simulink model "M03_Cascaded_ActiveYaw"  (R2025b)
settings: Solver=VariableStepAuto  StartTime=0.0  StopTime=t_sim_stop  RelTol=1e-3
undefined symbols (not defined in the file): a, b, g, k, L, mass, mu, P_gains, path_waypoints, v_ref_array, Vx_breakpoints
libraries: simulink x2, autolibshared x1
settings Model: Creator=Legion  LastModifiedBy=Legion

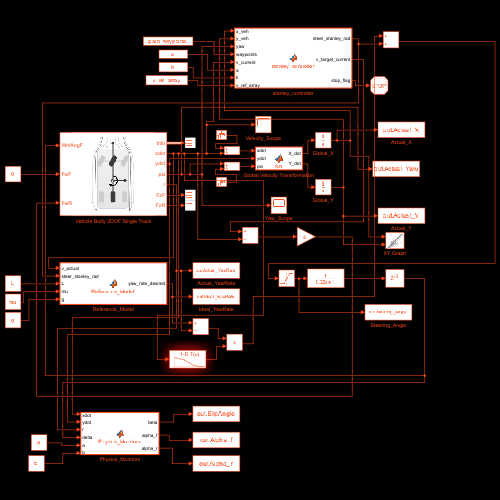
[thumbnail: Simulink's stored preview of the top-level diagram]
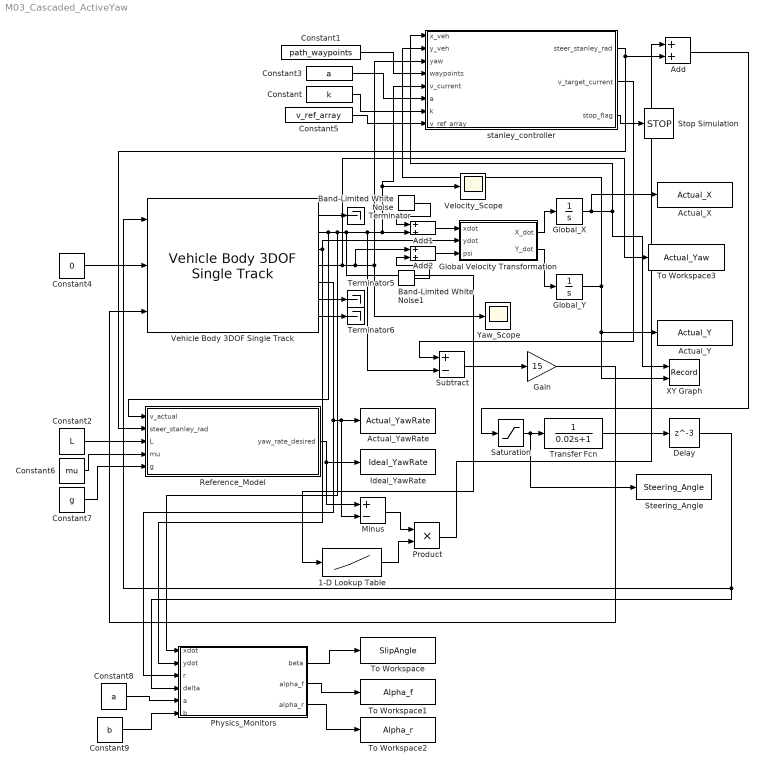
== system M03_Cascaded_ActiveYaw ==
  1-D Lookup Table : Lookup_n-D  NumberOfTableDimensions=1  BreakpointsForDimension1=Vx_breakpoints  Table=P_gains  InternalRulePriority=Speed  RndMeth=Simplest
  Actual_X : ToWorkspace  VariableName=Actual_X  SaveFormat=Timeseries  SampleTime=-1
  Actual_Y : ToWorkspace  VariableName=Actual_Y  SaveFormat=Timeseries  SampleTime=-1
  Actual_YawRate : ToWorkspace  VariableName=Actual_YawRate  SaveFormat=Timeseries  SampleTime=-1
  Add : Sum
  Add1 : Sum
  Add2 : Sum
  Band-Limited White Noise : simulink/Sources/Band-Limited White Noise  Cov=[0.0001]  Ts=0.01  seed=[23341]
  Band-Limited White Noise1 : simulink/Sources/Band-Limited White Noise  Cov=[0.0005]  Ts=0.01  seed=[23341]
  Constant : Constant  Value=k
  Constant1 : Constant  Value=path_waypoints
  Constant2 : Constant  Value=L
  Constant3 : Constant  Value=a
  Constant4 : Constant  Value=0
  Constant5 : Constant  Value=v_ref_array
  Constant6 : Constant  Value=mu
  Constant7 : Constant  Value=g
  Constant8 : Constant  Value=a
  Constant9 : Constant  Value=b
  Delay : Delay  DelayLength=3
  Gain : Gain  Gain=15
  Global Velocity Transformation : MATLAB Function  TreatAsAtomicUnit=on
  Global_X : Integrator  InitialCondition=path_waypoints(1,1)
  Global_Y : Integrator  InitialCondition=path_waypoints(1,2)
  Ideal_YawRate : ToWorkspace  VariableName=Ideal_YawRate  SaveFormat=Timeseries  SampleTime=-1
  Minus : Sum  Inputs=+-
  Physics_Monitors : MATLAB Function  TreatAsAtomicUnit=on
  Product : Product
  Reference_Model : MATLAB Function  TreatAsAtomicUnit=on
  Saturation : Saturate  UpperLimit=30 * pi/180  LowerLimit=-30 * pi/180
  Steering_Angle : ToWorkspace  VariableName=Steering_Angle  SaveFormat=Timeseries  SampleTime=-1
  Stop Simulation : Stop
  Subtract : Sum  Inputs=+-
  Terminator : Terminator
  Terminator5 : Terminator
  Terminator6 : Terminator
  To Workspace : ToWorkspace  VariableName=SlipAngle  SaveFormat=Timeseries  SampleTime=-1
  To Workspace1 : ToWorkspace  VariableName=Alpha_f  SaveFormat=Timeseries  SampleTime=-1
  To Workspace2 : ToWorkspace  VariableName=Alpha_r  SaveFormat=Timeseries  SampleTime=-1
  To Workspace3 : ToWorkspace  VariableName=Actual_Yaw  SaveFormat=Timeseries  SampleTime=-1
  Transfer Fcn : TransferFcn  Denominator=[0.02 1]
  Vehicle Body 3DOF Single Track : autolibshared/Vehicle Body 3DOF Single Track  trackMode=Single (bicycle)  inputMode=External longitudinal forces  frontSteerMode=on  rearSteerMode=off  windMode=off  muMode=off  extFMode=off  extMMode=off  htchFMode=off  htchMMode=off  extXo=off  extpsio=off  extxdoto=off  extro=off  extYo=off  extTamb=off  extydoto=off  aMode=2  NF=2  NR=2  m=mass  a=a  b=b  h=h  dh=1  hh=0.2  X_o=0  xdot_o=0.01  CalphaMode=off  sigmaMode=off  d=0  hl=0  w=[1.4,1.4]  Cy_f=Cy_f  Cy_r=Cy_r  sigma_f=.1  sigma_r=.1  alpha_f_brk=[-0.785, -0.628, -0.471, -0.314, -0.157, 0.000, 0.157, 0.314, 0.471, 0.628, 0.785]  Cy_f_data=[2000, 3000, 4000, 5500, 7000, 9000, 7000, 5500, 4000, 3000, 2000]  alpha_r_brk=[-0.785, -0.628, -0.471, -0.314, -0.157, 0.000, 0.157, 0.314, 0.471, 0.628, 0.785]  Cy_r_data=[2000, 3000, 4000, 5500, 7000, 9000, 7000, 5500, 4000, 3000, 2000]  Y_o=0  ydot_o=0  Izz=Izz  psi_o=atan2(path_waypoints(2,2)-path_waypoints(1,2), path_waypoints(2,1)-path_waypoints(1,1))  r_o=0  Af=Af  Cd=.3  Cl=.1  Cpm=.1  beta_w=[0 0.01:0.01:0.3]  Cs=[0 0.01:0.01:0.3]  Cym=[0 1e-6:0.01:0.3]  Pabs=101325  Tair=273  g=9.81  mu=mu  xdot_tol=.01  Fznom=Fznom  Fxtire_sat=7e4  Fytire_sat=7e4  longOff=0  latOff=0  vertOff=0  wrapAng=off
  Velocity_Scope : Scope
      settings: ActiveDisplayYMinimum=0.7024131164666485  ActiveDisplayYMaximum=1.4316639746586821
  XY Graph : Record  NumPorts=2.0  FileSettingsInternal="{\"entries\":[{\"content\":{\"excelSettings\":{\"content\":{},\"type\":\"Streamout.ExcelSettings\"},\"parquetSettings\":{\"content\":{},\"type\":\"Streamout.ParquetSettings\"}},\"type\":\"Streamout.FileSettingStorage\",\"uuid\":\"\"}],\"packageUris\":[\"http:\\/\\/schema.mathworks.com\\/mf0\\/streamout_blocks\\/R2020a\"],\"version\":\"1.0\"}"  FrameSettings=[0, 0]  Layout=[1 1]  SignalsInternal="{\"entries\":[{\"content\":{\"signals\":[{\"content\":{\"blockPath\":[],\"dimensions\":[1],\"domain\":\"\",\"lineColor\":\"#7e2f8e\",\"lineWidth\":2,\"port\":1,\"sid\":[\"\"],\"signalID\":1,\"signalName\":\"Global_X\"},\"type\":\"RecordBlkView.Signal\",\"uuid\":\"\"},{\"content\":{\"blockPath\":[],\"dimensions\":[1],\"domain\":\"\",\"lineColor\":\"#77ac30\",\"lineWidth\":2,\"port\":2,\"sid\":[\"\"],\"signalID\":2,\"signalName\":\"Global_Y\"},\"type\":\"RecordBlkView.Signal\",\"uuid\":\"\"}]},\"type\":\"RecordBlkView.InputSignals\",\"uuid\":\"\"}],\"packageUris\":[\"http:\\/\\/schema.mathworks.com\\/mf0\\/streamout_blocks\\/R2020a\"],\"version\":\"1.0\"}"  VisualizationBindings="{\"xyplotplugin\":{\"info\":[{\"series\":[],\"subplotID\":1}]}}"  CompatibilityTag=XY
  Yaw_Scope : Scope
      settings: ActiveDisplayYMinimum=-0.24426851447788056  ActiveDisplayYMaximum=1.1237341178679363
  stanley_controller : MATLAB Function  TreatAsAtomicUnit=on
  wires:
  Constant1/1 -> stanley_controller/4(waypoints)
  Subtract/1 -> Gain/1
  Gain/1 -> Vehicle Body 3DOF Single Track/3
  Vehicle Body 3DOF Single Track/3 -> Physics_Monitors/2(ydot), Global Velocity Transformation/2(ydot)
  stanley_controller/1(steer_stanley_rad) -> Add/2, Reference_Model/2(steer_stanley_rad)
  Vehicle Body 3DOF Single Track/7 -> Terminator6/1
  Vehicle Body 3DOF Single Track/2 -> Reference_Model/1(v_actual), Physics_Monitors/1(xdot), 1-D Lookup Table/1, Add1/2, stanley_controller/5(v_current), Velocity_Scope/1, Subtract/2
  Saturation/1 -> Steering_Angle/1, Transfer Fcn/1
  Constant3/1 -> stanley_controller/6(a)
  Vehicle Body 3DOF Single Track/1 -> Terminator/1
  Vehicle Body 3DOF Single Track/4 -> To Workspace3/1, Add2/1, stanley_controller/3(yaw), Yaw_Scope/1
  Global Velocity Transformation/2(Y_dot) -> Global_Y/1
  Transfer Fcn/1 -> Delay/1
  Global_Y/1 -> XY Graph/2, Actual_Y/1, stanley_controller/2(y_veh)
  Reference_Model/1(yaw_rate_desired) -> Minus/1, Ideal_YawRate/1
  Global Velocity Transformation/1(X_dot) -> Global_X/1
  Global_X/1 -> Actual_X/1, stanley_controller/1(x_veh), XY Graph/1
  Constant4/1 -> Vehicle Body 3DOF Single Track/2
  Vehicle Body 3DOF Single Track/6 -> Terminator5/1
  Vehicle Body 3DOF Single Track/5 -> Physics_Monitors/3(r), Actual_YawRate/1, Minus/2
  stanley_controller/2(v_target_current) -> Subtract/1
  Constant5/1 -> stanley_controller/8(v_ref_array)
  Constant/1 -> stanley_controller/7(k)
  Add/1 -> Saturation/1
  Constant2/1 -> Reference_Model/3(L)
  Constant7/1 -> Reference_Model/5(g)
  Constant6/1 -> Reference_Model/4(mu)
  Minus/1 -> Product/1
  1-D Lookup Table/1 -> Product/2
  Product/1 -> Add/1
  Physics_Monitors/3(alpha_r) -> To Workspace2/1
  Physics_Monitors/2(alpha_f) -> To Workspace1/1
  Physics_Monitors/1(beta) -> To Workspace/1
  Constant8/1 -> Physics_Monitors/5(a)
  Constant9/1 -> Physics_Monitors/6(b)
  stanley_controller/3(stop_flag) -> Stop Simulation/1
  Add1/1 -> Global Velocity Transformation/1(xdot)
  Add2/1 -> Global Velocity Transformation/3(psi)
  Band-Limited White Noise/1 -> Add1/1
  Band-Limited White Noise1/1 -> Add2/2
  Delay/1 -> Physics_Monitors/4(delta), Vehicle Body 3DOF Single Track/1

== matlab function M03_Cascaded_ActiveYaw/stanley_controller ==
  settings: updateMethod=DISCRETE
  data: x_veh input; steer_stanley_rad output; y_veh input; yaw input; waypoints input; v_current input; a input; k input; v_target_current output; v_ref_array input; stop_flag output
function [steer_stanley_rad, v_target_current, stop_flag] = stanley_controller(x_veh, y_veh, yaw, waypoints, v_current, a, k, v_ref_array)
    persistent has_finished last_closest_idx;
    if isempty(has_finished), has_finished = false; end
    if isempty(last_closest_idx), last_closest_idx = 1; end
    
    stop_flag = 0; % Default to not stopping
    
    % 1. The Finish Line Logic
    if last_closest_idx > (length(waypoints) * 0.95)
        dx_track = waypoints(end, 1) - waypoints(end-1, 1);
        dy_track = waypoints(end, 2) - waypoints(end-1, 2);
        dx_car = x_veh - waypoints(end, 1);
        dy_car = y_veh - waypoints(end, 2);
        if (dx_track * dx_car + dy_track * dy_car) > 0
            has_finished = true;
        end
    end
    
    if has_finished
        steer_stanley_rad = 0; v_target_current = 0; stop_flag = 1; 
        return; 
    end
    
    % 2. Project CG to Front Axle
    x_fa = x_veh + a * cos(yaw);
    y_fa = y_veh + a * sin(yaw);
    
    % 3. Find Closest Waypoint to Front Axle
    min_dist = inf; closest_idx = last_closest_idx;
    for i = last_closest_idx:(size(waypoints, 1) - 1)
        d = sqrt((waypoints(i,1) - x_fa)^2 + (waypoints(i,2) - y_fa)^2);
        if d < min_dist
            min_dist = d; closest_idx = i;
        end
    end
    last_closest_idx = closest_idx; 
    v_target_current = v_ref_array(closest_idx);
    
    % 4. Path Heading (yaw_path)
    dx = waypoints(closest_idx+1, 1) - waypoints(closest_idx, 1);
    dy = waypoints(closest_idx+1, 2) - waypoints(closest_idx, 2);
    yaw_path = atan2(dy, dx);
    
    % 5. Heading Error (psi_e)
    psi_e = yaw_path - yaw;
    psi_e = atan2(sin(psi_e), cos(psi_e));
    
    % 6. Cross-Track Error (e_fa) via Orthogonal Projection
    path_vec_x = dx; path_vec_y = dy;
    car_vec_x = x_fa - waypoints(closest_idx, 1);
    car_vec_y = y_fa - waypoints(closest_idx, 2);
    
    l2 = path_vec_x^2 + path_vec_y^2;
    if l2 > 0
        t = (car_vec_x * path_vec_x + car_vec_y * path_vec_y) / l2;
        t = max(0, min(1, t));
        proj_x = waypoints(closest_idx, 1) + t * path_vec_x;
        proj_y = waypoints(closest_idx, 2) + t * path_vec_y;
    else
        proj_x = waypoints(closest_idx, 1); proj_y = waypoints(closest_idx, 2);
    end
    
    e_fa_mag = sqrt((x_fa - proj_x)^2 + (y_fa - proj_y)^2);
    cross_prod = path_vec_x * (y_fa - waypoints(closest_idx, 2)) - path_vec_y * (x_fa - waypoints(closest_idx, 1));
    e_fa = -sign(cross_prod) * e_fa_mag;
    
    % 7. The Stanley Control Law
    k_soft = 0.1; 
    steer_stanley_rad = psi_e + atan((k * e_fa) / (v_current + k_soft));
    
    % 8. Physical Steering Limit (+/- 30 degrees)
    steer_max = 30 * (pi/180); 
    if steer_stanley_rad > steer_max, steer_stanley_rad = steer_max;
    elseif steer_stanley_rad < -steer_max, steer_stanley_rad = -steer_max; end
end

== matlab function M03_Cascaded_ActiveYaw/Global Velocity Transformation ==
  data: xdot input; X_dot output; ydot input; psi input; Y_dot output
function [X_dot, Y_dot] = fcn(xdot, ydot, psi)
    % Rotate Body Velocities into Global Map Velocities
    X_dot = xdot * cos(psi) - ydot * sin(psi);
    Y_dot = xdot * sin(psi) + ydot * cos(psi);
end

== matlab function M03_Cascaded_ActiveYaw/Reference_Model ==
  data: v_actual input; yaw_rate_desired output; steer_stanley_rad input; L input; mu input; g input
function yaw_rate_desired = Reference_Model(v_actual, steer_stanley_rad, L, mu, g)
    % 1. Prevent division by zero at standstill
    v_safe = max(v_actual, 0.1);
    
    % 2. Kinematic desired yaw rate (The Geometric Request)
    yaw_kinematic = (v_safe / L) * tan(steer_stanley_rad);
    
    % 3. Kamm Friction Circle Dynamic Limit (The Physical Reality)
    % Centripetal force limit: max yaw rate = (mu * g) / V
    yaw_max = (mu * g) / v_safe;
    
    % 4. The Interceptor (Clamp the request to the physical limit)
    if yaw_kinematic > yaw_max
        yaw_rate_desired = yaw_max;
    elseif yaw_kinematic < -yaw_max
        yaw_rate_desired = -yaw_max;
    else
        yaw_rate_desired = yaw_kinematic;
    end
end

== matlab function M03_Cascaded_ActiveYaw/Physics_Monitors ==
  data: xdot input; beta output; ydot input; r input; delta input; a input; b input; alpha_f output; alpha_r output
function [beta, alpha_f, alpha_r] = Physics_Monitors(xdot, ydot, r, delta, a, b)
    % This block mathematically derives the slip angles to prove tire saturation.
    % xdot: Longitudinal velocity (m/s)
    % ydot: Lateral velocity (m/s)
    % r: Yaw rate (rad/s)
    % delta: Actual front wheel steering angle (rad)
    % a, b: Distances from CG to front/rear axles (m)

    % 1. Safety limit to prevent division by zero when starting from a standstill
    v_x_safe = max(xdot, 0.1); 

    % 2. Vehicle Slip Angle (\beta)
    % Angle between the vehicle's longitudinal axis and its actual direction of travel
    beta = atan(ydot / v_x_safe);

    % 3. Front Tire Slip Angle (\alpha_f)
    % Combines lateral velocity, yaw rotation effect (a*r), and subtracts steering angle
    alpha_f = atan((ydot + a * r) / v_x_safe) - delta;

    % 4. Rear Tire Slip Angle (\alpha_r)
    % Combines lateral velocity and yaw rotation effect (rear axle moves opposite to front during yaw)
    alpha_r = atan((ydot - b * r) / v_x_safe);
end
